simulink model "TEST_LIDAR"  (R2022b)
settings: Solver=FixedStepAuto  StartTime=0.0  StopTime=inf  FixedStep=1e-3  RelTol=1e-3  EnableMultiTasking=on
model workspace (MAT data in the model file):
  SL_ROS_VariableLengthArrays_MaxSizes : object (value not decoded)
values from neighbouring files (symbols this model uses):
  data = theClient.GetLastFrameOfData()    [FuncMotive.m]
undefined symbols (not defined in the file or in its folder): angular, carstamp, CIRCUIT, CLTF_DAMP, CLTF_FREQ, CLTF_GAIN, CONTROL, CONTROL_INI, DiscIntNeverNeededParam, INPUT, linear, MCP3201, MD25, MODEL, MODEL_INI, mpcstate, MPU60X0, MPU9250, MSG, NAV_MPC_CONTROL, OUTPUT, RCRX, SAMPLING_TIME, SYSID_INPUT, VL6180X
libraries: raspberrypiCommlib x160, simulink x89, raspberrypiNetworklib x22, ros2lib x14, dspsigattribs x14, embedlinuxBasiclib x12, ctrlSharedLib x2, mpclib x1, vrlib x1, sldrtlib x1
(part 5 of 19)

== system TEST_LIDAR/MONITORING/COMMUNICATIONS/MSG_RX ==
  Enable : EnablePort
  Data Store Read : DataStoreRead  DataStoreName=MSG  SampleTime=SAMPLING_TIME  IndexOptions=Index vector (dialog)  Indices=1  OutputSizes=1
  Data Store Read2 : DataStoreRead  DataStoreName=CONTROL  SampleTime=SAMPLING_TIME  IndexOptions=Index vector (dialog)  Indices=1  OutputSizes=1
  Data Store Write1 : DataStoreWrite  DataStoreName=MSG  SampleTime=SAMPLING_TIME  IndexOptions=Index vector (dialog)  Indices=1  OutputSizes=1
  Data Store Write2 : DataStoreWrite  DataStoreName=CONTROL  SampleTime=SAMPLING_TIME  IndexOptions=Index vector (dialog)  Indices=1  OutputSizes=1
  MSG DECODER : MATLAB Function  Priority=20  TreatAsAtomicUnit=on
  wires:
  Data Store Read2/1 -> MSG DECODER/2(CONTROL_IN)
  MSG DECODER/1(MSG) -> Data Store Write1/1
  Data Store Read/1 -> MSG DECODER/1(MSG_IN)
  MSG DECODER/2(CONTROL) -> Data Store Write2/1

== system TEST_LIDAR/MONITORING/COMMUNICATIONS/MSG_TX  ==
  Enable : EnablePort
  Data Store Read : DataStoreRead  DataStoreName=MSG  SampleTime=SAMPLING_TIME  IndexOptions=Index vector (dialog)  Indices=1  OutputSizes=1
  Data Store Read6 : DataStoreRead  DataStoreName=CONTROL  SampleTime=SAMPLING_TIME  IndexOptions=Index vector (dialog)  Indices=1  OutputSizes=1
  Data Store Write1 : DataStoreWrite  DataStoreName=MSG  SampleTime=SAMPLING_TIME  IndexOptions=Index vector (dialog)  Indices=1  OutputSizes=1
  MSG CODER : MATLAB Function  Priority=20  TreatAsAtomicUnit=on
  wires:
  Data Store Read/1 -> MSG CODER/1(MSG_IN)
  MSG CODER/1(MSG) -> Data Store Write1/1
  Data Store Read6/1 -> MSG CODER/2(CONTROL)

== system TEST_LIDAR/MONITORING/ROS_COM/DYNAMICS PUBLISHERS ==
  Blank Message : ros2lib/Blank Message  messageClass=Message  entityType=geometry_msgs/Twist  messageType=geometry_msgs/Twist  SampleTime=-1
  Bus Assignment : BusAssignment  AssignedSignals=linear.x,linear.y,linear.z,angular.x,angular.y,angular.z
  Constant{,1..3} (4 alike) : Constant  Value=0  SampleTime=SAMPLING_TIME
  Data Store Read : DataStoreRead  DataStoreName=MODEL  SampleTime=SAMPLING_TIME  DataStoreElements=MODEL.OUTPUT.FORWARD_VEL#MODEL.OUTPUT.YAW_RATE  IndexOptions=Index vector (dialog)  Indices=1  OutputSizes=1
  Data Type Conversion4 : DataTypeConversion  SaturateOnIntegerOverflow=off  RndMeth=Floor
  Data Type Conversion9 : DataTypeConversion  SaturateOnIntegerOverflow=off  RndMeth=Floor
  Gain : Gain  Gain=-1
  POSE SCOPE : Scope  NumInputPorts=2
  Publish : ros2lib/Publish  topicSource=Specify your own  topic=/cmd_vel  messageType=geometry_msgs/Twist  QOSHistory=Keep last  QOSDepth=1  QOSReliability=Reliable  QOSDurability=Volatile
  wires:
  Constant1/1 -> Bus Assignment/4
  [CAR_YR] -> Gain/1
  Constant2/1 -> Bus Assignment/5
  [CAR_FV] -> Data Type Conversion4/1
  Data Store Read/2 -> [CAR_YR]
  Bus Assignment/1 -> Publish/1
  [CAR_FV] -> POSE SCOPE/1  "FV"
  Constant3/1 -> Bus Assignment/6
  Data Type Conversion4/1 -> Bus Assignment/2
  Data Type Conversion9/1 -> Bus Assignment/7
  [CAR_YR] -> POSE SCOPE/2  "YR"
  Blank Message/1 -> Bus Assignment/1
  Data Store Read/1 -> [CAR_FV]
  Constant/1 -> Bus Assignment/3
  Gain/1 -> Data Type Conversion9/1

== system TEST_LIDAR/MONITORING/SIMULATION: SCOPES/Second-order LPF 1 ==
  In : Inport
  Discrete Transfer Fcn : DiscreteTransferFcn  Numerator=Fd.num{1}  Denominator=Fd.den{1}  SampleTime=ts
  Out : Outport  VectorParamsAs1DForOutWhenUnconnected=off
  wires:
  In/1 -> Discrete Transfer Fcn/1
  Discrete Transfer Fcn/1 -> Out/1

== system TEST_LIDAR/MONITORING/SIMULATION: SCOPES/Second-order LPF 2 ==
  In : Inport
  Discrete Transfer Fcn : DiscreteTransferFcn  Numerator=Fd.num{1}  Denominator=Fd.den{1}  SampleTime=ts
  Out : Outport  VectorParamsAs1DForOutWhenUnconnected=off
  wires:
  In/1 -> Discrete Transfer Fcn/1
  Discrete Transfer Fcn/1 -> Out/1

== system TEST_LIDAR/MONITORING/SIMULATION: SCOPES/Second-order LPF 3 ==
  In : Inport
  Discrete Transfer Fcn : DiscreteTransferFcn  Numerator=Fd.num{1}  Denominator=Fd.den{1}  SampleTime=ts
  Out : Outport  VectorParamsAs1DForOutWhenUnconnected=off
  wires:
  In/1 -> Discrete Transfer Fcn/1
  Discrete Transfer Fcn/1 -> Out/1

== system TEST_LIDAR/MONITORING/SIMULATION: SCOPES/Second-order LPF 4 ==
  In : Inport
  Discrete Transfer Fcn : DiscreteTransferFcn  Numerator=Fd.num{1}  Denominator=Fd.den{1}  SampleTime=ts
  Out : Outport  VectorParamsAs1DForOutWhenUnconnected=off
  wires:
  In/1 -> Discrete Transfer Fcn/1
  Discrete Transfer Fcn/1 -> Out/1

== system TEST_LIDAR/MONITORING/SIMULATION: SCOPES/Second-order LPF 5 ==
  In : Inport
  Discrete Transfer Fcn : DiscreteTransferFcn  Numerator=Fd.num{1}  Denominator=Fd.den{1}  SampleTime=ts
  Out : Outport  VectorParamsAs1DForOutWhenUnconnected=off
  wires:
  In/1 -> Discrete Transfer Fcn/1
  Discrete Transfer Fcn/1 -> Out/1

== system TEST_LIDAR/SIMULATION/RC TRANSMITTER /SWB ==
  UP : Inport
  DOWN : Inport  Port=2
  Constant1 : Constant  Value=1500  SampleTime=-1
  Gain : Gain  Gain=-500
  Gain5 : Gain  Gain=500
  Sum : Sum  Inputs=3
  SWITCH : Outport
  wires:
  Constant1/1 -> Sum/2
  Sum/1 -> SWITCH/1
  UP/1 -> Gain/1
  Gain5/1 -> Sum/3
  Gain/1 -> Sum/1
  DOWN/1 -> Gain5/1

== system TEST_LIDAR/SIMULATION/RC TRANSMITTER /SWC ==
  UP : Inport
  DOWN : Inport  Port=2
  Constant1 : Constant  Value=1500  SampleTime=-1
  Gain : Gain  Gain=-500
  Gain5 : Gain  Gain=500
  Sum : Sum  Inputs=3
  SWITCH : Outport
  wires:
  DOWN/1 -> Gain5/1
  Gain/1 -> Sum/1
  Gain5/1 -> Sum/3
  UP/1 -> Gain/1
  Sum/1 -> SWITCH/1
  Constant1/1 -> Sum/2

== system TEST_LIDAR/SIMULATION/READ IMU/ LPF 3 ==
  IN : Inport
  ALFA : Inport  Port=2  SampleTime=MPU60X0.SAMPLING_TIME
  Bias : Bias  Bias=single(1)  SaturateOnIntegerOverflow=off
  Gain : Gain  Gain=-1
  Product : Product
  Product2 : Product
  Sum : Sum  Inputs=|++
  Unit Delay : UnitDelay  SampleTime=-1  HasFrameUpgradeWarning=on
  OUT : Outport  VectorParamsAs1DForOutWhenUnconnected=off
  wires:
  IN/1 -> Product2/1
  Bias/1 -> Product2/2
  Product2/1 -> Sum/1
  Gain/1 -> Bias/1
  ALFA/1 -> Product/2, Gain/1
  Sum/1 -> OUT/1, Unit Delay/1
  Product/1 -> Sum/2
  Unit Delay/1 -> Product/1

== system TEST_LIDAR/SIMULATION/READ IMU/ LPF 4 ==
  IN : Inport
  ALFA : Inport  Port=2  SampleTime=MPU60X0.SAMPLING_TIME
  Bias : Bias  Bias=single(1)  SaturateOnIntegerOverflow=off
  Gain : Gain  Gain=-1
  Product : Product
  Product2 : Product
  Sum : Sum  Inputs=|++
  Unit Delay : UnitDelay  SampleTime=-1  HasFrameUpgradeWarning=on
  OUT : Outport  VectorParamsAs1DForOutWhenUnconnected=off
  wires:
  IN/1 -> Product2/1
  Bias/1 -> Product2/2
  Product2/1 -> Sum/1
  Gain/1 -> Bias/1
  ALFA/1 -> Product/2, Gain/1
  Sum/1 -> OUT/1, Unit Delay/1
  Product/1 -> Sum/2
  Unit Delay/1 -> Product/1

== system TEST_LIDAR/SIMULATION/READ IMU/FILTER POLE ==
  Constant : Constant  Value=MPU60X0.SAMPLING_TIME  OutDataTypeStr=single  SampleTime=MPU60X0.SAMPLING_TIME
  Data Store Read4 : DataStoreRead  DataStoreName=CONTROL  SampleTime=MPU60X0.SAMPLING_TIME  DataStoreElements=CONTROL.PARAM.IMU_FILT_FREQ  IndexOptions=Index vector (dialog)  Indices=1  OutputSizes=1
  Gain : Gain  Gain=-2*pi
  Math Function : Math  SignedPower=on
  Product1 : Product
  ALFA : Outport  VectorParamsAs1DForOutWhenUnconnected=off
  wires:
  Data Store Read4/1 -> Gain/1
  Product1/1 -> Math Function/1
  Constant/1 -> Product1/1
  Math Function/1 -> ALFA/1
  Gain/1 -> Product1/2

== system TEST_LIDAR/SIMULATION/READ IMU/LPF 1 ==
  IN : Inport
  ALFA : Inport  Port=2  SampleTime=MPU60X0.SAMPLING_TIME
  Bias : Bias  Bias=single(1)  SaturateOnIntegerOverflow=off
  Gain : Gain  Gain=-1
  Product : Product
  Product2 : Product
  Sum : Sum  Inputs=|++
  Unit Delay : UnitDelay  InitialCondition=[CONTROL_INI.PARAM.GRAVITY*CONTROL_INI.STATE.VEHICLE_MODE ; 0 ; -CONTROL_INI.PARAM.GRAVITY*(1-CONTROL_INI.STATE.VEHICLE_MODE)]  SampleTime=-1  HasFrameUpgradeWarning=on
  OUT : Outport  VectorParamsAs1DForOutWhenUnconnected=off
  wires:
  Unit Delay/1 -> Product/1
  Product/1 -> Sum/2
  Sum/1 -> Unit Delay/1, OUT/1
  ALFA/1 -> Gain/1, Product/2
  Gain/1 -> Bias/1
  Product2/1 -> Sum/1
  Bias/1 -> Product2/2
  IN/1 -> Product2/1

== system TEST_LIDAR/SIMULATION/READ IMU/LPF 2 2 ==
  IN : Inport
  ALFA : Inport  Port=2  SampleTime=MPU60X0.SAMPLING_TIME
  Bias : Bias  Bias=single(1)  SaturateOnIntegerOverflow=off
  Gain : Gain  Gain=-1
  Product : Product
  Product2 : Product
  Sum : Sum  Inputs=|++
  Unit Delay : UnitDelay  InitialCondition=[CONTROL_INI.PARAM.GRAVITY*CONTROL_INI.STATE.VEHICLE_MODE ; 0 ; -CONTROL_INI.PARAM.GRAVITY*(1-CONTROL_INI.STATE.VEHICLE_MODE)]  SampleTime=-1  HasFrameUpgradeWarning=on
  OUT : Outport  VectorParamsAs1DForOutWhenUnconnected=off
  wires:
  Unit Delay/1 -> Product/1
  Product/1 -> Sum/2
  Sum/1 -> Unit Delay/1, OUT/1
  ALFA/1 -> Gain/1, Product/2
  Gain/1 -> Bias/1
  Product2/1 -> Sum/1
  Bias/1 -> Product2/2
  IN/1 -> Product2/1

== system TEST_LIDAR/GAZEBO SIMULATION/COMMUNICATIONS/TCP//IP/MSG_RX ==
  Bus Assignment : BusAssignment  AssignedSignals=RX_BUFFER
  Bus Selector : BusSelector  OutputSignals=data
  Data Store Read : DataStoreRead  DataStoreName=MSG  IndexOptions=Index vector (dialog)  Indices=1  OutputSizes=1
  Data Store Write1 : DataStoreWrite  DataStoreName=MSG  IndexOptions=Index vector (dialog)  Indices=1  OutputSizes=1
  Subscribe : ros2lib/Subscribe  topicSource=Specify your own  topic=/pc_to_car  messageType=time_custom_msgs/Tiempos  sampleTime=SAMPLING_TIME  QOSHistory=Keep last  QOSDepth=1  QOSReliability=Reliable  QOSDurability=Volatile
      settings: LibrarySourceBlock=roslib/ROS 2/Subscribe
  Terminator : Terminator
  OutROSmsg : Outport
  wires:
  Bus Selector/1 -> Bus Assignment/2  "<data>"
  Data Store Read/1 -> Bus Assignment/1
  Bus Assignment/1 -> Data Store Write1/1
  Subscribe/2 -> OutROSmsg/1, Bus Selector/1
  Subscribe/1 -> Terminator/1

== system TEST_LIDAR/GAZEBO SIMULATION/COMMUNICATIONS/TCP//IP/MSG_TX ==
  InROSmsg : Inport
  Enable : EnablePort
  Bus Assignment : BusAssignment  AssignedSignals=data,carstamp
  Current Time : ros2lib/Current Time  OutputFormat=bus  SampleTime=-1  ModelName=CAR_CONTROL_SYSTEM
      settings: LibrarySourceBlock=roslib/ROS 2/Current Time
  Data Store Read1 : DataStoreRead  DataStoreName=MSG  SampleTime=SAMPLING_TIME  DataStoreElements=MSG.TX_BUFFER(:,1)  IndexOptions=Index vector (dialog)  Indices=1  OutputSizes=1
  Publish : ros2lib/Publish  topicSource=Specify your own  topic=/car_to_pc  messageType=time_custom_msgs/Tiempos  QOSHistory=Keep last  QOSDepth=1  QOSReliability=Reliable  QOSDurability=Volatile
      settings: LibrarySourceBlock=roslib/ROS 2/Publish
  wires:
  Data Store Read1/1 -> Bus Assignment/2
  InROSmsg/1 -> Bus Assignment/1
  Bus Assignment/1 -> Publish/1
  Current Time/1 -> Bus Assignment/3

== system TEST_LIDAR/GAZEBO SIMULATION/COMMUNICATIONS/UART/MSG_RX ==
  Data Store Write : DataStoreWrite  DataStoreName=CONTROL  DataStoreElements=CONTROL.STATE.CURRENT_STATUS_PC#CONTROL.STATE.PC_BUTTON#CONTROL.STATE.PC_LIMIT_SWITCH(:,:)  IndexOptions=Index vector (dialog)  Indices=1  OutputSizes=1
  Demux : Demux  Outputs=[1 1 4]
  Serial Read : raspberrypiCommlib/Serial Read  board=Pi 3 Model B+  SCIModule_=/dev/ttyS0  Baudrate_=57600  Parity=None  StopBits_=1  HardwareFlowControl=None  ByteOrder=LittleEndian  DataLength=6  DataType=uint8  OutputStatus=on  SampleTime=SAMPLING_TIME  blockPlatform=RaspberryPi
  Terminator1 : Terminator
  wires:
  Serial Read/2 -> Terminator1/1
  Serial Read/1 -> Demux/1
  Demux/1 -> Data Store Write/1
  Demux/2 -> Data Store Write/2
  Demux/3 -> Data Store Write/3

== system TEST_LIDAR/GAZEBO SIMULATION/COMMUNICATIONS/UART/MSG_TX ==
  Enable : EnablePort
  Data Store Read : DataStoreRead  DataStoreName=CONTROL  SampleTime=SAMPLING_TIME  DataStoreElements=CONTROL.STATE.CURRENT_STATUS_SYS  IndexOptions=Index vector (dialog)  Indices=1  OutputSizes=1
  Serial Write : raspberrypiCommlib/Serial Write  board=Pi 3 Model B+  SCIModule_=/dev/ttyS0  Baudrate_=57600  Parity=None  StopBits_=1  HardwareFlowControl=None  ByteOrder=LittleEndian  OutputStatus=off  blockPlatform=RaspberryPi
  wires:
  Data Store Read/1 -> Serial Write/1

== system TEST_LIDAR/GAZEBO SIMULATION/COMMUNICATIONS/UART_MUX/BT MCS ==
  Data : Inport
  Enable : EnablePort
  Data Store Read2 : DataStoreRead  DataStoreName=CONTROL  SampleTime=10e-03  IndexOptions=Index vector (dialog)  Indices=1  OutputSizes=1
  Data Store Write2 : DataStoreWrite  DataStoreName=CONTROL  SampleTime=10e-03  IndexOptions=Index vector (dialog)  Indices=1  OutputSizes=1
  MCS RX : MATLAB Function  Priority=20  TreatAsAtomicUnit=on
  wires:
  Data Store Read2/1 -> MCS RX/1(CONTROL_IN)
  MCS RX/1(CONTROL) -> Data Store Write2/1
  Data/1 -> MCS RX/2(BUFFER_RX_LAST)

== system TEST_LIDAR/GAZEBO SIMULATION/COMMUNICATIONS/UART_MUX/RCRX iBUS ==
  Data : Inport
  Enable : EnablePort
  BUS UPDATE : MATLAB Function  Priority=20  TreatAsAtomicUnit=on
  Constant : Constant  Value=RCRX  SampleTime=SAMPLING_TIME
  Data Store Read19 : DataStoreRead  DataStoreName=CONTROL  SampleTime=SAMPLING_TIME  IndexOptions=Index vector (dialog)  Indices=1  OutputSizes=1
  Data Store Write1 : DataStoreWrite  DataStoreName=CONTROL  IndexOptions=Index vector (dialog)  Indices=1  OutputSizes=1
  Display : Display
  Display3 : Display
  MATLAB Function : MATLAB Function  TreatAsAtomicUnit=on
  wires:
  MATLAB Function/1(CH_RAW) -> Display/1, BUS UPDATE/2(CH_RAW)
  BUS UPDATE/1(CONTROL) -> Data Store Write1/1
  Data Store Read19/1 -> BUS UPDATE/1(CONTROL_IN)
  Data/1 -> Display3/1, MATLAB Function/1(iBUS_DATA)
  Constant/1 -> BUS UPDATE/3(RCRX)

== system TEST_LIDAR/GAZEBO SIMULATION/COMMUNICATIONS/UDP//ROS/MSG_RX ==
  Bus Assignment : BusAssignment  AssignedSignals=RX_BUFFER
  Data Store Read : DataStoreRead  DataStoreName=MSG  IndexOptions=Index vector (dialog)  Indices=1  OutputSizes=1
  Data Store Write1 : DataStoreWrite  DataStoreName=MSG  IndexOptions=Index vector (dialog)  Indices=1  OutputSizes=1
  Terminator1 : Terminator
  UDP Receive : raspberrypiNetworklib/UDP Receive  localURL='0.0.0.0'  localPort=25000  remoteURL='0.0.0.0'  remotePort=-1  recvBufferSize=8192  signalDatatype=uint8  dims=255  isVarSize=off  showBlockingTime=off  blockingTime=0  sampletime=0.01  blockPlatform=Raspberry Pi
  wires:
  UDP Receive/1 -> Bus Assignment/2
  Data Store Read/1 -> Bus Assignment/1
  Bus Assignment/1 -> Data Store Write1/1
  UDP Receive/2 -> Terminator1/1

== system TEST_LIDAR/GAZEBO SIMULATION/COMMUNICATIONS/UDP//ROS/MSG_TX ==
  Enable : EnablePort
  Data Store Read1 : DataStoreRead  DataStoreName=MSG  SampleTime=SAMPLING_TIME  DataStoreElements=MSG.TX_BUFFER(:,1)  IndexOptions=Index vector (dialog)  Indices=1  OutputSizes=1
  UDP Send : raspberrypiNetworklib/UDP Send  remoteURL='255.255.255.255'  remotePort=25000  localURL='0.0.0.0'  localPortSource=Automatically determine  localPort=-1  sampletime=-1  blockPlatform=Raspberry Pi  separateLengthPort=0
  wires:
  Data Store Read1/1 -> UDP Send/1

== system TEST_LIDAR/GAZEBO SIMULATION/SENSORS/READ IMU/ LPF 3 ==
  IN : Inport
  ALFA : Inport  Port=2  SampleTime=SAMPLING_TIME
  Bias : Bias  Bias=1  SaturateOnIntegerOverflow=off
  Gain : Gain  Gain=-1
  Product : Product
  Product2 : Product
  Sum : Sum  Inputs=|++
  Unit Delay : UnitDelay  SampleTime=-1  HasFrameUpgradeWarning=on
  OUT : Outport  VectorParamsAs1DForOutWhenUnconnected=off
  wires:
  IN/1 -> Product2/1
  Bias/1 -> Product2/2
  Product2/1 -> Sum/1
  Gain/1 -> Bias/1
  ALFA/1 -> Product/2, Gain/1
  Sum/1 -> OUT/1, Unit Delay/1
  Product/1 -> Sum/2
  Unit Delay/1 -> Product/1

== system TEST_LIDAR/GAZEBO SIMULATION/SENSORS/READ IMU/ LPF 4 ==
  IN : Inport
  ALFA : Inport  Port=2  SampleTime=SAMPLING_TIME
  Bias : Bias  Bias=1  SaturateOnIntegerOverflow=off
  Gain : Gain  Gain=-1
  Product : Product
  Product2 : Product
  Sum : Sum  Inputs=|++
  Unit Delay : UnitDelay  SampleTime=-1  HasFrameUpgradeWarning=on
  OUT : Outport  VectorParamsAs1DForOutWhenUnconnected=off
  wires:
  IN/1 -> Product2/1
  Bias/1 -> Product2/2
  Product2/1 -> Sum/1
  Gain/1 -> Bias/1
  ALFA/1 -> Product/2, Gain/1
  Sum/1 -> OUT/1, Unit Delay/1
  Product/1 -> Sum/2
  Unit Delay/1 -> Product/1

== system TEST_LIDAR/GAZEBO SIMULATION/SENSORS/READ IMU/FILTER POLE ==
  Constant : Constant  Value=SAMPLING_TIME  OutDataTypeStr=single  SampleTime=SAMPLING_TIME
  Data Store Read4 : DataStoreRead  DataStoreName=CONTROL  SampleTime=MPU60X0.SAMPLING_TIME  DataStoreElements=CONTROL.PARAM.IMU_FILT_FREQ  IndexOptions=Index vector (dialog)  Indices=1  OutputSizes=1
  Gain : Gain  Gain=-2*pi
  Math Function : Math  SignedPower=on
  Product1 : Product
  ALFA : Outport  VectorParamsAs1DForOutWhenUnconnected=off
  wires:
  Data Store Read4/1 -> Gain/1
  Product1/1 -> Math Function/1
  Constant/1 -> Product1/1
  Math Function/1 -> ALFA/1
  Gain/1 -> Product1/2

== system TEST_LIDAR/GAZEBO SIMULATION/SENSORS/READ IMU/LPF 1 ==
  IN : Inport
  ALFA : Inport  Port=2  SampleTime=SAMPLING_TIME
  Bias : Bias  Bias=1  SaturateOnIntegerOverflow=off
  Gain : Gain  Gain=-1
  Product : Product
  Product2 : Product
  Sum : Sum  Inputs=|++
  Unit Delay : UnitDelay  InitialCondition=[CONTROL_INI.PARAM.GRAVITY*CONTROL_INI.STATE.VEHICLE_MODE ; 0 ; -CONTROL_INI.PARAM.GRAVITY*(1-CONTROL_INI.STATE.VEHICLE_MODE)]  SampleTime=-1  HasFrameUpgradeWarning=on
  OUT : Outport  VectorParamsAs1DForOutWhenUnconnected=off
  wires:
  Unit Delay/1 -> Product/1
  Product/1 -> Sum/2
  Sum/1 -> Unit Delay/1, OUT/1
  ALFA/1 -> Gain/1, Product/2
  Gain/1 -> Bias/1
  Product2/1 -> Sum/1
  Bias/1 -> Product2/2
  IN/1 -> Product2/1

== system TEST_LIDAR/GAZEBO SIMULATION/SENSORS/READ IMU/LPF 2  ==
  IN : Inport
  ALFA : Inport  Port=2  SampleTime=SAMPLING_TIME
  Bias : Bias  Bias=1  SaturateOnIntegerOverflow=off
  Gain : Gain  Gain=-1
  Product : Product
  Product2 : Product
  Sum : Sum  Inputs=|++
  Unit Delay : UnitDelay  InitialCondition=[CONTROL_INI.PARAM.GRAVITY*CONTROL_INI.STATE.VEHICLE_MODE ; 0 ; -CONTROL_INI.PARAM.GRAVITY*(1-CONTROL_INI.STATE.VEHICLE_MODE)]  SampleTime=-1  HasFrameUpgradeWarning=on
  OUT : Outport  VectorParamsAs1DForOutWhenUnconnected=off
  wires:
  Unit Delay/1 -> Product/1
  Product/1 -> Sum/2
  Sum/1 -> Unit Delay/1, OUT/1
  ALFA/1 -> Gain/1, Product/2
  Gain/1 -> Bias/1
  Product2/1 -> Sum/1
  Bias/1 -> Product2/2
  IN/1 -> Product2/1

== system TEST_LIDAR/GAZEBO SIMULATION/SENSORS/WALL RANGE SENSOR/ANGLE AND DISTANCE COMPUTATION ==
  Data Store Read : DataStoreRead  DataStoreName=FRONT_DISTANCE  SampleTime=SAMPLING_TIME  IndexOptions=Index vector (dialog)  Indices=1  OutputSizes=1
  Data Store Read1 : DataStoreRead  DataStoreName=REAR_DISTANCE  IndexOptions=Index vector (dialog)  Indices=1  OutputSizes=1
  Data Store Read2 : DataStoreRead  DataStoreName=CONTROL  SampleTime=SAMPLING_TIME  IndexOptions=Index vector (dialog)  Indices=1  OutputSizes=1
  Data Store Write1 : DataStoreWrite  DataStoreName=CONTROL  IndexOptions=Index vector (dialog)  Indices=1  OutputSizes=1
  YAW_ANGLE_DISTANCE_COMPUTATION : MATLAB Function  TreatAsAtomicUnit=on
  wires:
  Data Store Read/1 -> YAW_ANGLE_DISTANCE_COMPUTATION/1(FRONT_DISTANCE)
  Data Store Read1/1 -> YAW_ANGLE_DISTANCE_COMPUTATION/2(REAR_DISTANCE)
  Data Store Read2/1 -> YAW_ANGLE_DISTANCE_COMPUTATION/3(CONTROL_IN)
  YAW_ANGLE_DISTANCE_COMPUTATION/1(CONTROL) -> Data Store Write1/1

== system TEST_LIDAR/GAZEBO SIMULATION/SENSORS/WALL RANGE SENSOR/FRONT ==
  Bus Selector : BusSelector  OutputSignals=ranges
  Data Store Write : DataStoreWrite  DataStoreName=FRONT_DISTANCE  IndexOptions=Index vector (dialog)  Indices=1  OutputSizes=1
  Data Type Conversion : DataTypeConversion  OutDataTypeStr=double  SaturateOnIntegerOverflow=off  RndMeth=Floor
  Subscribe : ros2lib/Subscribe  topicSource=Select from ROS network  topic=/front_dist_sensor  messageType=sensor_msgs/LaserScan  sampleTime=SAMPLING_TIME  QOSHistory=Keep last  QOSDepth=1  QOSReliability=Reliable  QOSDurability=Volatile
      settings: LibrarySourceBlock=roslib/ROS 2/Subscribe
  Terminator : Terminator
  wires:
  Bus Selector/1 -> Data Type Conversion/1  "<ranges>"
  Data Type Conversion/1 -> Data Store Write/1
  Subscribe/2 -> Bus Selector/1
  Subscribe/1 -> Terminator/1

== system TEST_LIDAR/GAZEBO SIMULATION/SENSORS/WALL RANGE SENSOR/REAR ==
  Bus Selector : BusSelector  OutputSignals=ranges
  Data Store Write : DataStoreWrite  DataStoreName=REAR_DISTANCE  IndexOptions=Index vector (dialog)  Indices=1  OutputSizes=1
  Data Type Conversion : DataTypeConversion  OutDataTypeStr=double  SaturateOnIntegerOverflow=off  RndMeth=Floor
  Subscribe : ros2lib/Subscribe  topicSource=Select from ROS network  topic=/back_dist_sensor  messageType=sensor_msgs/LaserScan  sampleTime=SAMPLING_TIME  QOSHistory=Keep last  QOSDepth=1  QOSReliability=Reliable  QOSDurability=Volatile
      settings: LibrarySourceBlock=roslib/ROS 2/Subscribe
  Terminator : Terminator
  wires:
  Data Type Conversion/1 -> Data Store Write/1
  Subscribe/2 -> Bus Selector/1
  Subscribe/1 -> Terminator/1
  Bus Selector/1 -> Data Type Conversion/1  "<ranges>"

== system TEST_LIDAR/HARDWARE/ACTUATORS/MD25_I2C/MD25 INITIALIZATION ==
  Enable : EnablePort
  Compare To Zero{,1..4} (5 alike) : simulink/Logic and Bit Operations/Compare To Zero  relop===  OutDataTypeStr=boolean
  Constant1 : Constant  Value=MD25.MODE_BYTE  OutDataTypeStr=uint8  SampleTime=SAMPLING_TIME
  Constant10 : Constant  Value=hex2dec('32')  OutDataTypeStr=uint8  SampleTime=SAMPLING_TIME
  Constant2 : Constant  Value=hex2dec('10')  OutDataTypeStr=uint8  SampleTime=SAMPLING_TIME
  Constant3 : Constant  Value=MD25.MODE_BYTE  OutDataTypeStr=uint8  SampleTime=SAMPLING_TIME
  Constant6 : Constant  Value=hex2dec('20')  OutDataTypeStr=uint8  SampleTime=SAMPLING_TIME
  Constant9 : Constant  Value=hex2dec('30')  OutDataTypeStr=uint8  SampleTime=SAMPLING_TIME
  Data Store Write2 : DataStoreWrite  DataStoreName=MD25_INIT  IndexOptions=Index vector (dialog)  Indices=1  OutputSizes=1
  Logical Operator : Logic  Priority=100  Inputs=6  AllPortsSameDT=off  OutDataTypeStr=boolean
  MD25.ACCEL_RATE : raspberrypiCommlib/I2C Master Write  Priority=30  BoardProperty=Pi 3 Model B+  Mode=Master  SlaveAddress=MD25.ADDRESS  SlaveByteOrder=BigEndian  Direction=Transmitter  RegisterAddressMode=on  RegisterAddress=MD25.ACCEL_RATE  SlaveDataType=uint8  DataLength=1  NoAck=off  RepeatedStart=off  OutputStatus=on
  MD25.COMMAND 1 : raspberrypiCommlib/I2C Master Write  Priority=10  BoardProperty=Pi 3 Model B+  Mode=Master  SlaveAddress=MD25.ADDRESS  SlaveByteOrder=BigEndian  Direction=Transmitter  RegisterAddressMode=on  RegisterAddress=MD25.COMMAND  SlaveDataType=uint8  DataLength=1  NoAck=off  RepeatedStart=off  OutputStatus=on
  MD25.COMMAND 2 : raspberrypiCommlib/I2C Master Write  Priority=20  BoardProperty=Pi 3 Model B+  Mode=Master  SlaveAddress=MD25.ADDRESS  SlaveByteOrder=BigEndian  Direction=Transmitter  RegisterAddressMode=on  RegisterAddress=MD25.COMMAND  SlaveDataType=uint8  DataLength=1  NoAck=off  RepeatedStart=off  OutputStatus=on
  MD25.COMMAND 3 : raspberrypiCommlib/I2C Master Write  Priority=30  BoardProperty=Pi 3 Model B+  Mode=Master  SlaveAddress=MD25.ADDRESS  SlaveByteOrder=BigEndian  Direction=Transmitter  RegisterAddressMode=on  RegisterAddress=MD25.COMMAND  SlaveDataType=uint8  DataLength=1  NoAck=off  RepeatedStart=off  OutputStatus=on
  MD25.MODE : raspberrypiCommlib/I2C Master Write  Priority=0  BoardProperty=Pi 3 Model B+  Mode=Master  SlaveAddress=MD25.ADDRESS  SlaveByteOrder=BigEndian  Direction=Transmitter  RegisterAddressMode=on  RegisterAddress=MD25.MODE  SlaveDataType=uint8  DataLength=1  NoAck=off  RepeatedStart=off  OutputStatus=on
  MD25.MODE READ : raspberrypiCommlib/I2C Master Read  Priority=40  BoardProperty=Pi 3 Model B+  Mode=Master  SlaveAddress=MD25.ADDRESS  SlaveByteOrder=BigEndian  Direction=Receiver  RegisterAddressMode=on  RegisterAddress=MD25.MODE  SlaveDataType=uint8  DataLength=uint8(1)  NoAck=off  RepeatedStart=off  OutputStatus=off  SampleTime=SAMPLING_TIME
  Relational Operator : RelationalOperator  Operator===  OutDataTypeStr=boolean  RndMeth=Simplest  InputSameDT=off
  wires:
  MD25.MODE/1 -> Compare To Zero/1
  Constant3/1 -> MD25.MODE/1
  MD25.COMMAND 1/1 -> Compare To Zero1/1
  Constant6/1 -> MD25.COMMAND 1/1
  MD25.COMMAND 2/1 -> Compare To Zero2/1
  Constant9/1 -> MD25.COMMAND 2/1
  Compare To Zero/1 -> Logical Operator/1
  Compare To Zero1/1 -> Logical Operator/2
  Compare To Zero2/1 -> Logical Operator/3
  Constant10/1 -> MD25.COMMAND 3/1
  MD25.COMMAND 3/1 -> Compare To Zero3/1
  Compare To Zero3/1 -> Logical Operator/4
  Logical Operator/1 -> Data Store Write2/1
  MD25.MODE READ/1 -> Relational Operator/1
  Constant1/1 -> Relational Operator/2
  Relational Operator/1 -> Logical Operator/6
  MD25.ACCEL_RATE/1 -> Compare To Zero4/1
  Constant2/1 -> MD25.ACCEL_RATE/1
  Compare To Zero4/1 -> Logical Operator/5

== system TEST_LIDAR/HARDWARE/ACTUATORS/MD25_I2C/READ BATTERY VOLTAGE ==
  Enable : EnablePort
  BATTERY VOLTAGE FILTER : MATLAB Function  Priority=30  TreatAsAtomicUnit=on
  Constant1 : Constant  Value=MD25.THR_NLFILT  VectorParams1D=off  OutDataTypeStr=double  SampleTime=SAMPLING_TIME
  Constant2 : Constant  Value=MD25.ALFA_FILT  VectorParams1D=off  OutDataTypeStr=double  SampleTime=SAMPLING_TIME
  Constant3 : Constant  Value=MD25.BATTERY_VOLT  VectorParams1D=off  OutDataTypeStr=double  SampleTime=SAMPLING_TIME
  Data Store Read : DataStoreRead  DataStoreName=CONTROL  SampleTime=SAMPLING_TIME  IndexOptions=Index vector (dialog)  Indices=1  OutputSizes=1
  Data Store Write : DataStoreWrite  DataStoreName=CONTROL  IndexOptions=Index vector (dialog)  Indices=1  OutputSizes=1
  Data Type Conversion1 : DataTypeConversion  OutDataTypeStr=double  SaturateOnIntegerOverflow=off  RndMeth=Floor
  Gain : Gain  Gain=0.1
  MD25.BATTERY_VOLTS : raspberrypiCommlib/I2C Master Read  Priority=10  BoardProperty=Pi 3 Model B+  Mode=Master  SlaveAddress=MD25.ADDRESS  SlaveByteOrder=BigEndian  Direction=Receiver  RegisterAddressMode=on  RegisterAddress=MD25.BATTERY_VOLTS  SlaveDataType=uint8  DataLength=uint8(1)  NoAck=off  RepeatedStart=off  OutputStatus=off  SampleTime=SAMPLING_TIME
  wires:
  Data Store Read/1 -> BATTERY VOLTAGE FILTER/1(CONTROL_IN)
  BATTERY VOLTAGE FILTER/1(CONTROL) -> Data Store Write/1
  MD25.BATTERY_VOLTS/1 -> Data Type Conversion1/1
  Data Type Conversion1/1 -> Gain/1
  Gain/1 -> BATTERY VOLTAGE FILTER/2(BATTERY_VOLT)
  Constant3/1 -> BATTERY VOLTAGE FILTER/3(RATED_BATTERY_VOLT)
  Constant1/1 -> BATTERY VOLTAGE FILTER/4(THR_NLFILT)
  Constant2/1 -> BATTERY VOLTAGE FILTER/5(ALFA_FILT)

== system TEST_LIDAR/HARDWARE/ACTUATORS/MD25_I2C/READ MOTOR CURRENT ==
  Enable : EnablePort
  Bus Assignment : BusAssignment  AssignedSignals=INPUT.MOTOR_CURRENT
  Data Store Read : DataStoreRead  DataStoreName=CONTROL  SampleTime=SAMPLING_TIME  IndexOptions=Index vector (dialog)  Indices=1  OutputSizes=1
  Data Store Write : DataStoreWrite  DataStoreName=CONTROL  IndexOptions=Index vector (dialog)  Indices=1  OutputSizes=1
  Data Type Conversion1 : DataTypeConversion  OutDataTypeStr=double  SaturateOnIntegerOverflow=off  RndMeth=Floor
  Gain : Gain  Gain=0.1
  MD25.MOTOR1_CURRENT : raspberrypiCommlib/I2C Master Read  Priority=10  BoardProperty=Pi 3 Model B+  Mode=Master  SlaveAddress=MD25.ADDRESS  SlaveByteOrder=BigEndian  Direction=Receiver  RegisterAddressMode=on  RegisterAddress=MD25.MOTOR1_CURRENT  SlaveDataType=uint8  DataLength=uint8(2)  NoAck=off  RepeatedStart=off  OutputStatus=off  SampleTime=SAMPLING_TIME
  wires:
  Data Store Read/1 -> Bus Assignment/1
  Bus Assignment/1 -> Data Store Write/1
  Data Type Conversion1/1 -> Gain/1
  Gain/1 -> Bus Assignment/2
  MD25.MOTOR1_CURRENT/1 -> Data Type Conversion1/1

== system TEST_LIDAR/HARDWARE/ACTUATORS/MD25_I2C/READ MOTOR ENCODER ==
  Enable : EnablePort
  Data Store Read : DataStoreRead  DataStoreName=CONTROL  SampleTime=SAMPLING_TIME  IndexOptions=Index vector (dialog)  Indices=1  OutputSizes=1
  Data Store Write1 : DataStoreWrite  DataStoreName=CONTROL  IndexOptions=Index vector (dialog)  Indices=1  OutputSizes=1
  MD25.ENC1A : raspberrypiCommlib/I2C Master Read  Priority=10  BoardProperty=Pi 3 Model B+  Mode=Master  SlaveAddress=MD25.ADDRESS  SlaveByteOrder=BigEndian  Direction=Receiver  RegisterAddressMode=on  RegisterAddress=MD25.ENC1A  SlaveDataType=uint8  DataLength=uint8(8)  NoAck=off  RepeatedStart=off  OutputStatus=off  SampleTime=SAMPLING_TIME
  READ ENCODER ANGLE : MATLAB Function  Commented=on  TreatAsAtomicUnit=on
  READ_ENCODER : MATLAB Function  TreatAsAtomicUnit=on
  READ_ENCODER OLD : MATLAB Function  Commented=on  TreatAsAtomicUnit=on
  wires:
  Data Store Read/1 -> READ_ENCODER/1(CONTROL_IN)
  READ_ENCODER/1(CONTROL) -> Data Store Write1/1
  MD25.ENC1A/1 -> READ_ENCODER/2(MOTOR_ENC_BYTES)

== system TEST_LIDAR/HARDWARE/ACTUATORS/MD25_I2C/RESET MOTOR ENCODER ==
  Enable : EnablePort
  Constant6 : Constant  Value=hex2dec('20')  OutDataTypeStr=uint8  SampleTime=SAMPLING_TIME
  MD25.COMMAND 1 : raspberrypiCommlib/I2C Master Write  BoardProperty=Pi 3 Model B+  Mode=Master  SlaveAddress=MD25.ADDRESS  SlaveByteOrder=BigEndian  Direction=Transmitter  RegisterAddressMode=on  RegisterAddress=MD25.COMMAND  SlaveDataType=uint8  DataLength=1  NoAck=off  RepeatedStart=off  OutputStatus=off
  wires:
  Constant6/1 -> MD25.COMMAND 1/1

== system TEST_LIDAR/HARDWARE/ACTUATORS/MD25_I2C/WRITE PWM MOTOR  ==
  Enable : EnablePort
  Bus Assignment : BusAssignment  AssignedSignals=OUTPUT.MOTOR_PWM
  Constant2 : Constant  Commented=on  Value=hex2dec('10')  OutDataTypeStr=uint8  SampleTime=SAMPLING_TIME
  Constant5 : Constant  Value=MD25.PWM_MAX  OutDataTypeStr=double  SampleTime=SAMPLING_TIME
  Constant6 : Constant  Value=MD25.PWM_MIN  OutDataTypeStr=double  SampleTime=SAMPLING_TIME
  Data Store Read1 : DataStoreRead  DataStoreName=CONTROL  SampleTime=SAMPLING_TIME  IndexOptions=Index vector (dialog)  Indices=1  OutputSizes=1
  Data Store Read2 : DataStoreRead  DataStoreName=CONTROL  SampleTime=SAMPLING_TIME  IndexOptions=Index vector (dialog)  Indices=1  OutputSizes=1
  Data Store Write1 : DataStoreWrite  DataStoreName=CONTROL  IndexOptions=Index vector (dialog)  Indices=1  OutputSizes=1
  Demux : Demux  Outputs=2
  MD25.ACCEL_RATE : raspberrypiCommlib/I2C Master Write  Priority=0  Commented=on  BoardProperty=Pi 3 Model B+  Mode=Master  SlaveAddress=MD25.ADDRESS  SlaveByteOrder=BigEndian  Direction=Transmitter  RegisterAddressMode=on  RegisterAddress=MD25.ACCEL_RATE  SlaveDataType=uint8  DataLength=1  NoAck=off  RepeatedStart=off  OutputStatus=off
  MD25.SPEED1 : raspberrypiCommlib/I2C Master Write  BoardProperty=Pi 3 Model B+  Mode=Master  SlaveAddress=MD25.ADDRESS  SlaveByteOrder=BigEndian  Direction=Transmitter  RegisterAddressMode=on  RegisterAddress=MD25.SPEED1  SlaveDataType=uint8  DataLength=1  NoAck=off  RepeatedStart=off  OutputStatus=off
  MD25.SPEED2 : raspberrypiCommlib/I2C Master Write  BoardProperty=Pi 3 Model B+  Mode=Master  SlaveAddress=MD25.ADDRESS  SlaveByteOrder=BigEndian  Direction=Transmitter  RegisterAddressMode=on  RegisterAddress=MD25.SPEED2  SlaveDataType=uint8  DataLength=1  NoAck=off  RepeatedStart=off  OutputStatus=off
  PWM CONVERSION : MATLAB Function  TreatAsAtomicUnit=on
  wires:
  Constant5/1 -> PWM CONVERSION/2(PWM_MAX)
  Constant6/1 -> PWM CONVERSION/3(PWM_MIN)
  PWM CONVERSION/1(PWM_BYTE) -> Demux/1
  Data Store Read1/1 -> Bus Assignment/1
  Bus Assignment/1 -> Data Store Write1/1
  PWM CONVERSION/2(MOTOR_PWM) -> Bus Assignment/2
  Demux/2 -> MD25.SPEED1/1
  Demux/1 -> MD25.SPEED2/1
  Constant2/1 -> MD25.ACCEL_RATE/1
  Data Store Read2/1 -> PWM CONVERSION/1(CONTROL)

== system TEST_LIDAR/HARDWARE/COMMUNICATIONS/TCP//IP/MSG_RX ==
  Bus Assignment : BusAssignment  AssignedSignals=RX_BUFFER
  Data Store Read : DataStoreRead  DataStoreName=MSG  IndexOptions=Index vector (dialog)  Indices=1  OutputSizes=1
  Data Store Write1 : DataStoreWrite  DataStoreName=MSG  IndexOptions=Index vector (dialog)  Indices=1  OutputSizes=1
  TCP/IP Receive : raspberrypiNetworklib/TCP//IP Receive  Mode_=Server  LocalServerPort_=27001  RemoteAddr_=127.0.0.1  RemoteServerPort_=25000  DataType_=uint8  DataSize_=1400  SampleTime_=SAMPLING_TIME  SimulateUsing=Code generation  ClientPortBindingSelection_=off  ClientPortToBind_=35000  BlockingMode_=off  BlockTimeout_=0.1  BlockPlatform=RASPBERRYPI
  Terminator1 : Terminator
  wires:
  TCP/IP Receive/1 -> Bus Assignment/2
  Data Store Read/1 -> Bus Assignment/1
  Bus Assignment/1 -> Data Store Write1/1
  TCP/IP Receive/2 -> Terminator1/1

== system TEST_LIDAR/HARDWARE/COMMUNICATIONS/TCP//IP/MSG_TX ==
  Enable : EnablePort
  Data Store Read1 : DataStoreRead  DataStoreName=MSG  SampleTime=SAMPLING_TIME  DataStoreElements=MSG.TX_BUFFER(:,1)  IndexOptions=Index vector (dialog)  Indices=1  OutputSizes=1
  TCP/IP Send : raspberrypiNetworklib/TCP//IP Send  Mode_=Server  LocalServerPort_=27000  RemoteAddr_=127.0.0.1  RemoteServerPort_=25000  SimulateUsing=Code generation  ClientPortBindingSelection_=off  ClientPortToBind_=35000  BlockingMode_=off  BlockTimeout_=0.1  BlockPlatform=RASPBERRYPI
  wires:
  Data Store Read1/1 -> TCP/IP Send/1

== system TEST_LIDAR/HARDWARE/COMMUNICATIONS/UART/MSG_RX ==
  Data Store Write : DataStoreWrite  DataStoreName=CONTROL  DataStoreElements=CONTROL.STATE.CURRENT_STATUS_PC#CONTROL.STATE.PC_BUTTON#CONTROL.STATE.PC_LIMIT_SWITCH(:,:)  IndexOptions=Index vector (dialog)  Indices=1  OutputSizes=1
  Demux : Demux  Outputs=[1 1 4]
  Serial Read : raspberrypiCommlib/Serial Read  board=Pi 3 Model B+  SCIModule_=/dev/ttyS0  Baudrate_=57600  Parity=None  StopBits_=1  HardwareFlowControl=None  ByteOrder=LittleEndian  DataLength=6  DataType=uint8  OutputStatus=on  SampleTime=SAMPLING_TIME  blockPlatform=RaspberryPi
  Terminator1 : Terminator
  wires:
  Serial Read/2 -> Terminator1/1
  Serial Read/1 -> Demux/1
  Demux/1 -> Data Store Write/1
  Demux/2 -> Data Store Write/2
  Demux/3 -> Data Store Write/3

== system TEST_LIDAR/HARDWARE/COMMUNICATIONS/UART/MSG_TX ==
  Enable : EnablePort
  Data Store Read : DataStoreRead  DataStoreName=CONTROL  SampleTime=SAMPLING_TIME  DataStoreElements=CONTROL.STATE.CURRENT_STATUS_SYS  IndexOptions=Index vector (dialog)  Indices=1  OutputSizes=1
  Serial Write : raspberrypiCommlib/Serial Write  board=Pi 3 Model B+  SCIModule_=/dev/ttyS0  Baudrate_=57600  Parity=None  StopBits_=1  HardwareFlowControl=None  ByteOrder=LittleEndian  OutputStatus=off  blockPlatform=RaspberryPi
  wires:
  Data Store Read/1 -> Serial Write/1

== system TEST_LIDAR/HARDWARE/COMMUNICATIONS/UART_MUX/BT MCS ==
  Data : Inport
  Enable : EnablePort
  Data Store Read2 : DataStoreRead  DataStoreName=CONTROL  SampleTime=10e-03  IndexOptions=Index vector (dialog)  Indices=1  OutputSizes=1
  Data Store Write2 : DataStoreWrite  DataStoreName=CONTROL  SampleTime=10e-03  IndexOptions=Index vector (dialog)  Indices=1  OutputSizes=1
  MCS RX : MATLAB Function  Priority=20  TreatAsAtomicUnit=on
  wires:
  Data Store Read2/1 -> MCS RX/1(CONTROL_IN)
  MCS RX/1(CONTROL) -> Data Store Write2/1
  Data/1 -> MCS RX/2(BUFFER_RX_LAST)

== system TEST_LIDAR/HARDWARE/COMMUNICATIONS/UART_MUX/RCRX iBUS ==
  Data : Inport
  Enable : EnablePort
  BUS UPDATE : MATLAB Function  Priority=20  TreatAsAtomicUnit=on
  Constant : Constant  Value=RCRX  SampleTime=SAMPLING_TIME
  Data Store Read19 : DataStoreRead  DataStoreName=CONTROL  SampleTime=SAMPLING_TIME  IndexOptions=Index vector (dialog)  Indices=1  OutputSizes=1
  Data Store Write1 : DataStoreWrite  DataStoreName=CONTROL  IndexOptions=Index vector (dialog)  Indices=1  OutputSizes=1
  Display : Display
  Display3 : Display
  MATLAB Function : MATLAB Function  TreatAsAtomicUnit=on
  wires:
  MATLAB Function/1(CH_RAW) -> Display/1, BUS UPDATE/2(CH_RAW)
  BUS UPDATE/1(CONTROL) -> Data Store Write1/1
  Data Store Read19/1 -> BUS UPDATE/1(CONTROL_IN)
  Data/1 -> Display3/1, MATLAB Function/1(iBUS_DATA)
  Constant/1 -> BUS UPDATE/3(RCRX)

== system TEST_LIDAR/HARDWARE/COMMUNICATIONS/UDP//ROS/MSG_RX ==
  Bus Assignment : BusAssignment  AssignedSignals=RX_BUFFER
  Data Store Read : DataStoreRead  DataStoreName=MSG  IndexOptions=Index vector (dialog)  Indices=1  OutputSizes=1
  Data Store Write1 : DataStoreWrite  DataStoreName=MSG  IndexOptions=Index vector (dialog)  Indices=1  OutputSizes=1
  Terminator1 : Terminator
  UDP Receive : raspberrypiNetworklib/UDP Receive  localURL='0.0.0.0'  localPort=25000  remoteURL='0.0.0.0'  remotePort=-1  recvBufferSize=8192  signalDatatype=uint8  dims=255  isVarSize=off  showBlockingTime=off  blockingTime=0  sampletime=0.01  blockPlatform=Raspberry Pi
  wires:
  UDP Receive/1 -> Bus Assignment/2
  Data Store Read/1 -> Bus Assignment/1
  Bus Assignment/1 -> Data Store Write1/1
  UDP Receive/2 -> Terminator1/1

== system TEST_LIDAR/HARDWARE/COMMUNICATIONS/UDP//ROS/MSG_TX ==
  Enable : EnablePort
  Data Store Read1 : DataStoreRead  DataStoreName=MSG  SampleTime=SAMPLING_TIME  DataStoreElements=MSG.TX_BUFFER(:,1)  IndexOptions=Index vector (dialog)  Indices=1  OutputSizes=1
  UDP Send : raspberrypiNetworklib/UDP Send  remoteURL='255.255.255.255'  remotePort=25000  localURL='0.0.0.0'  localPortSource=Automatically determine  localPort=-1  sampletime=-1  blockPlatform=Raspberry Pi  separateLengthPort=0
  wires:
  Data Store Read1/1 -> UDP Send/1

== system TEST_LIDAR/HARDWARE/SENSORS/IMU MPU60X0_SPI/INITIALIZATION ==
  Enable : EnablePort
  Compare To Constant : simulink/Logic and Bit Operations/Compare To Constant  relop===  const=MPU60X0.CONFIG_BYTE  OutDataTypeStr=boolean
  Data Store Write : DataStoreWrite  DataStoreName=MPU60X0_INIT  IndexOptions=Index vector (dialog)  Indices=1  OutputSizes=1
  MPU9250.ACCEL_CONFIG : raspberrypiCommlib/SPI Register Write  Priority=50  BoardProperty=Pi 3 Model B+  SSPin=SPI0_CE1  SPIModule=uint32(0)  Mode=Master  BusSpeed=1000000  Pin=SPI0_CE0  FirstBitToTransfer=Most significant bit (MSB)  ClockMode=3  BlockFunction=Write  RegisterAddress=MPU60X0.ACCEL_CONFIG  OutputDataType=int8  OutputDataLength=1
  MPU9250.CONFIG : raspberrypiCommlib/SPI Register Write  Priority=80  BoardProperty=Pi 3 Model B+  SSPin=SPI0_CE1  SPIModule=uint32(0)  Mode=Master  BusSpeed=1000000  Pin=SPI0_CE0  FirstBitToTransfer=Most significant bit (MSB)  ClockMode=3  BlockFunction=Write  RegisterAddress=MPU60X0.CONFIG  OutputDataType=int8  OutputDataLength=1
  MPU9250.FIFO_EN : raspberrypiCommlib/SPI Register Write  Priority=70  BoardProperty=Pi 3 Model B+  SSPin=SPI0_CE1  SPIModule=uint32(0)  Mode=Master  BusSpeed=1000000  Pin=SPI0_CE0  FirstBitToTransfer=Most significant bit (MSB)  ClockMode=3  BlockFunction=Write  RegisterAddress=MPU60X0.FIFO_EN  OutputDataType=int8  OutputDataLength=1
  MPU9250.GYRO_CONFIG : raspberrypiCommlib/SPI Register Write  Priority=60  BoardProperty=Pi 3 Model B+  SSPin=SPI0_CE1  SPIModule=uint32(0)  Mode=Master  BusSpeed=1000000  Pin=SPI0_CE0  FirstBitToTransfer=Most significant bit (MSB)  ClockMode=3  BlockFunction=Write  RegisterAddress=MPU60X0.GYRO_CONFIG  OutputDataType=int8  OutputDataLength=1
  MPU9250.INT_ENABLE : raspberrypiCommlib/SPI Register Write  Priority=40  BoardProperty=Pi 3 Model B+  SSPin=SPI0_CE1  SPIModule=uint32(0)  Mode=Master  BusSpeed=1000000  Pin=SPI0_CE0  FirstBitToTransfer=Most significant bit (MSB)  ClockMode=3  BlockFunction=Write  RegisterAddress=MPU60X0.INT_ENABLE  OutputDataType=int8  OutputDataLength=1
  MPU9250.PWR_MGMT_1 : raspberrypiCommlib/SPI Register Write  Priority=20  BoardProperty=Pi 3 Model B+  SSPin=SPI0_CE1  SPIModule=uint32(0)  Mode=Master  BusSpeed=1000000  Pin=SPI0_CE0  FirstBitToTransfer=Most significant bit (MSB)  ClockMode=3  BlockFunction=Write  RegisterAddress=MPU60X0.PWR_MGMT_1  OutputDataType=int8  OutputDataLength=1
  MPU9250.SMPLRT_DIV : raspberrypiCommlib/SPI Register Write  Priority=30  BoardProperty=Pi 3 Model B+  SSPin=SPI0_CE1  SPIModule=uint32(0)  Mode=Master  BusSpeed=1000000  Pin=SPI0_CE0  FirstBitToTransfer=Most significant bit (MSB)  ClockMode=3  BlockFunction=Write  RegisterAddress=MPU60X0.SMPLRT_DIV  OutputDataType=int8  OutputDataLength=1
  MPU9250.USER_CTRL : raspberrypiCommlib/SPI Register Write  Priority=10  BoardProperty=Pi 3 Model B+  SSPin=SPI0_CE1  SPIModule=uint32(0)  Mode=Master  BusSpeed=1000000  Pin=SPI0_CE0  FirstBitToTransfer=Most significant bit (MSB)  ClockMode=3  BlockFunction=Write  RegisterAddress=MPU60X0.USER_CTRL  OutputDataType=int8  OutputDataLength=1
  OUT_X_L1 : Constant  Value=MPU60X0.CONFIG_BYTE  OutDataTypeStr=uint8  SampleTime=-1
  OUT_X_L2 : Constant  Value=MPU60X0.INT_ENABLE_BYTE  OutDataTypeStr=uint8  SampleTime=-1
  OUT_X_L21 : Constant  Value=MPU60X0.FIFO_EN_BYTE  OutDataTypeStr=uint8  SampleTime=-1
  OUT_X_L22 : Constant  Value=MPU60X0.USER_CTRL_BYTE  OutDataTypeStr=uint8  SampleTime=-1
  OUT_X_L23 : Constant  Value=MPU60X0.PWR_MGMT_1_BYTE  OutDataTypeStr=uint8  SampleTime=-1
  OUT_X_L24 : Constant  Value=MPU60X0.SMPLRT_DIV_BYTE  OutDataTypeStr=uint8  SampleTime=-1
  OUT_X_L8 : Constant  Value=MPU60X0.ACCEL_CONFIG_BYTE  OutDataTypeStr=uint8  SampleTime=-1
  OUT_X_L9 : Constant  Value=MPU60X0.GYRO_CONFIG_BYTE  OutDataTypeStr=uint8  SampleTime=-1
  Subsystem : Subsystem  Priority=90  mask{Register=MPU60X0.CONFIG, n=1}
      mask prompts: Register "MPU9250 Register"; n "Data size (bytes)"
  wires:
  Compare To Constant/1 -> Data Store Write/1
  Subsystem/1(Out1) -> Compare To Constant/1
  OUT_X_L8/1 -> MPU9250.ACCEL_CONFIG/1
  OUT_X_L23/1 -> MPU9250.PWR_MGMT_1/1
  OUT_X_L21/1 -> MPU9250.FIFO_EN/1
  OUT_X_L22/1 -> MPU9250.USER_CTRL/1
  OUT_X_L2/1 -> MPU9250.INT_ENABLE/1
  OUT_X_L9/1 -> MPU9250.GYRO_CONFIG/1
  OUT_X_L24/1 -> MPU9250.SMPLRT_DIV/1
  OUT_X_L1/1 -> MPU9250.CONFIG/1

== system TEST_LIDAR/HARDWARE/SENSORS/IMU MPU60X0_SPI/READ FIFO ==
  Enable : EnablePort
  Constant2 : Constant  Commented=on  Value=bin2dec('01000100');  OutDataTypeStr=uint8  SampleTime=SAMPLING_TIME
  Constant3 : Constant  Value=MPU60X0.ACCEL_SSF  SampleTime=SAMPLING_TIME
  Constant4 : Constant  Value=MPU60X0.GYRO_SSF  SampleTime=SAMPLING_TIME
  Constant7 : Constant  Value=MPU60X0.FIFO_LENGTH  OutDataTypeStr=uint8  SampleTime=SAMPLING_TIME
  Data Store Read : DataStoreRead  DataStoreName=CONTROL  DataStoreElements=CONTROL_BUS.INPUT.IMU.ACCEL_MEAN(:,:)#CONTROL_BUS.INPUT.IMU.GYRO_MEAN(:,:)  IndexOptions=Index vector (dialog)  Indices=1  OutputSizes=1
  Data Store Read2 : DataStoreRead  DataStoreName=CONTROL  SampleTime=SAMPLING_TIME  IndexOptions=Index vector (dialog)  Indices=1  OutputSizes=1
  Data Store Write : DataStoreWrite  DataStoreName=CONTROL  IndexOptions=Index vector (dialog)  Indices=1  OutputSizes=1
  Data Store Write1 : DataStoreWrite  DataStoreName=MPU60X0_RAW_GYRO_MEAN  IndexOptions=Index vector (dialog)  Indices=1  OutputSizes=1
  Data Store Write2 : DataStoreWrite  DataStoreName=MPU60X0_RAW_ACCEL_MEAN  IndexOptions=Index vector (dialog)  Indices=1  OutputSizes=1
  Data Type Conversion : DataTypeConversion  OutDataTypeStr=double  SaturateOnIntegerOverflow=off  RndMeth=Floor
  Data Type Conversion4 : DataTypeConversion  OutDataTypeStr=int16  SaturateOnIntegerOverflow=off  RndMeth=Floor
  EVEN POSITIONS : Selector  InputPortWidth=uint8(12*MPU9250.FIFO_LENGTH)  IndexOptions=Index vector (dialog)  Indices=2:2:uint8(12*MPU9250.FIFO_LENGTH)  OutputSizes=1
  FIFO READ : Subsystem  mask{Register=MPU60X0.FIFO_R_W, n=12*MPU60X0.FIFO_LENGTH}
      mask prompts: Register "MPU9250 Register"; n "Data size (bytes)"
      mask DialogControl Control2 Prompt: (Add text here)
  FIFO RESET : raspberrypiCommlib/SPI Register Write  Priority=20  Commented=on  BoardProperty=Pi 3 Model B+  SSPin=SPI0_CE1  SPIModule=uint32(0)  Mode=Master  BusSpeed=1000000  Pin=SPI0_CE0  FirstBitToTransfer=Most significant bit (MSB)  ClockMode=3  BlockFunction=Write  RegisterAddress=MPU60X0.USER_CTRL  OutputDataType=int8  OutputDataLength=1
  FIFO_PROCESSING : MATLAB Function  Priority=30  TreatAsAtomicUnit=on
  Gain61 : Gain  Gain=2^8
  Mux : Mux
  ODD POSITIONS : Selector  InputPortWidth=uint8(12*MPU9250.FIFO_LENGTH)  IndexOptions=Index vector (dialog)  Indices=1:2:uint8(12*MPU9250.FIFO_LENGTH)  OutputSizes=1
  Sum61 : Sum  Inputs=|++
  To File : ToFile  Filename=BLACK_BOX_FIFO.mat  MatrixName=FIFO_LOG
  wires:
  Data Store Read/2 -> Mux/4
  Data Store Read/1 -> Mux/3
  FIFO_PROCESSING/5(GYRO_FIFO) -> Mux/2
  FIFO_PROCESSING/4(ACCEL_FIFO) -> Mux/1
  Constant4/1 -> FIFO_PROCESSING/5(GYRO_SSF)
  Constant3/1 -> FIFO_PROCESSING/4(ACCEL_SSF)
  Mux/1 -> Data Type Conversion/1
  Data Type Conversion/1 -> To File/1
  Data Type Conversion4/1 -> FIFO_PROCESSING/2(FIFO_DATA)
  FIFO READ/1(Out1) -> ODD POSITIONS/1, EVEN POSITIONS/1
  FIFO_PROCESSING/3(RAW_ACCEL_MEAN_OUT) -> Data Store Write2/1
  FIFO_PROCESSING/2(RAW_GYRO_MEAN_OUT) -> Data Store Write1/1
  Constant2/1 -> FIFO RESET/1
  Data Store Read2/1 -> FIFO_PROCESSING/1(CONTROL_IN)
  Sum61/1 -> Data Type Conversion4/1
  FIFO_PROCESSING/1(CONTROL_OUT) -> Data Store Write/1
  Constant7/1 -> FIFO_PROCESSING/3(FIFO_LENGTH)
  EVEN POSITIONS/1 -> Sum61/2
  Gain61/1 -> Sum61/1
  ODD POSITIONS/1 -> Gain61/1
